simulink model "empty"  (R2018b)
settings: Solver=VariableStepAuto  StartTime=0.0  StopTime=10.0  RelTol=1e-3
settings Model: Creator=yangr  LastModifiedBy=yangr

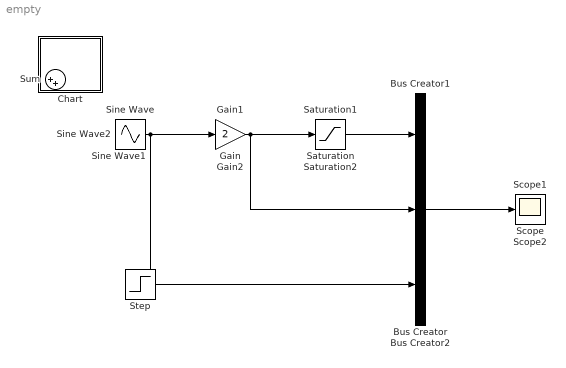
== system empty ==
  Bus Creator : BusCreator  Inputs=3
  Bus Creator1 : BusCreator  Inputs=3
  Bus Creator2 : BusCreator  Inputs=3
  Chart : Stateflow chart  TreatAsAtomicUnit=on
  Gain : Gain  Gain=2
  Gain1 : Gain  Gain=2
  Gain2 : Gain  Gain=2
  Saturation : Saturate
  Saturation1 : Saturate
  Saturation2 : Saturate
  Scope : Scope
  Scope1 : Scope
  Scope2 : Scope
  Sine Wave : Sin  SampleTime=0
  Sine Wave1 : Sin  SampleTime=0
  Sine Wave2 : Sin  SampleTime=0
  Step : Step  SampleTime=0
  Sum : Sum  Inputs=|++
  wires:
  Sine Wave/1 -> Gain/1, Bus Creator/3
  Gain/1 -> Saturation/1, Bus Creator/2
  Saturation/1 -> Bus Creator/1
  Bus Creator/1 -> Scope/1
  Sine Wave1/1 -> Gain1/1, Bus Creator1/3
  Gain1/1 -> Saturation1/1, Bus Creator1/2
  Saturation1/1 -> Bus Creator1/1
  Bus Creator1/1 -> Scope1/1
  Sine Wave2/1 -> Gain2/1, Bus Creator2/3
  Gain2/1 -> Saturation2/1, Bus Creator2/2
  Saturation2/1 -> Bus Creator2/1
  Bus Creator2/1 -> Scope2/1

== stateflow chart empty/Chart ==
